simulink subsystem "State_Estimation_2WD_NO_REGEN"  (R2023b)
settings: Solver=VariableStepAuto  StartTime=0.0  StopTime=10.0  RelTol=1e-3
undefined symbols (not defined in the file): nI
libraries: dspstat3 x1
settings Model: Creator=Inver  LastModifiedBy=Inver

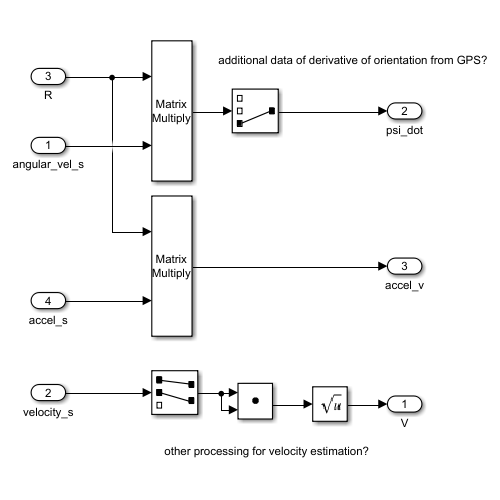
[thumbnail: Simulink's stored preview of the top-level diagram]
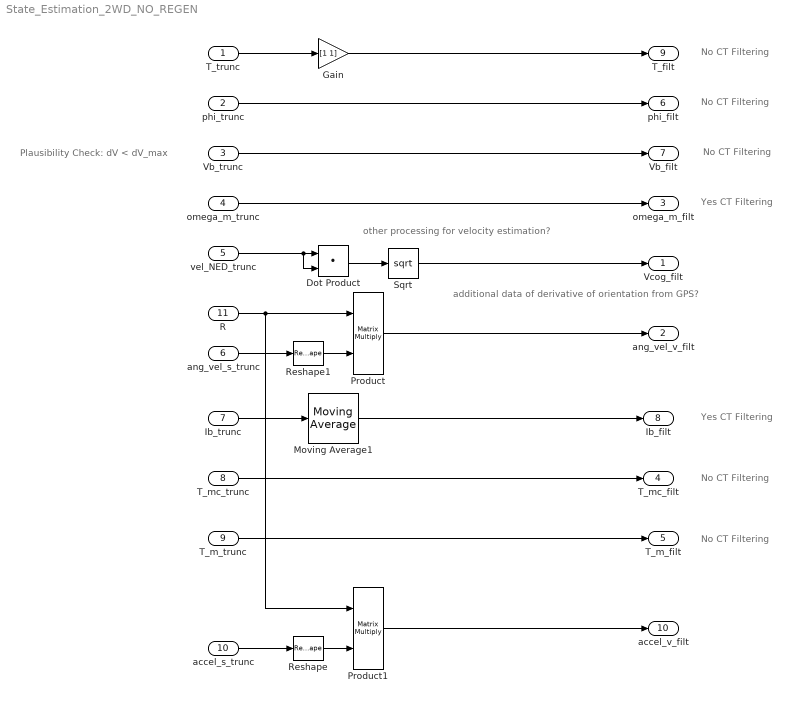
== system State_Estimation_2WD_NO_REGEN ==
  note: No CT Filtering
  note: Yes CT Filtering
  note: No CT Filtering
  note: No CT Filtering
  note: No CT Filtering
  note: No CT Filtering
  note: Plausibility Check: dV < dV_max
  note: Yes CT Filtering
  note: additional data of derivative of orientation from GPS?
  note: other processing for velocity estimation?
  T_trunc : Inport
  phi_trunc : Inport  Port=2
  Vb_trunc : Inport  Port=3
  omega_m_trunc : Inport  Port=4
  vel_NED_trunc : Inport  Port=5
  ang_vel_s_trunc : Inport  Port=6
  Ib_trunc : Inport  Port=7
  T_mc_trunc : Inport  Port=8
  T_m_trunc : Inport  Port=9
  accel_s_trunc : Inport  Port=10
  R : Inport  Port=11
  Dot Product : DotProduct  OutDataTypeStr=Inherit: Inherit via internal rule
  Gain : Gain  Gain=[1 1]
  Moving Average1 : dspstat3/Moving Average  Method=Sliding window  ForgettingFactorPort=off  SpecifyWindowLength=on  WindowLength=nI  OverlapLength=nI-1  AllowArbitraryInputLength=off  ForgettingFactor=0.9  SimulateUsing=Code generation
  Product : Product  Multiplication=Matrix(*)
  Product1 : Product  Multiplication=Matrix(*)
  Reshape : Reshape  OutputDimensions=[3 1]
  Reshape1 : Reshape  OutputDimensions=[3 1]
  Sqrt : Sqrt
  Vcog_filt : Outport
  ang_vel_v_filt : Outport  Port=2
  omega_m_filt : Outport  Port=3
  T_mc_filt : Outport  Port=4
  T_m_filt : Outport  Port=5
  phi_filt : Outport  Port=6
  Vb_filt : Outport  Port=7
  Ib_filt : Outport  Port=8
  T_filt : Outport  Port=9
  accel_v_filt : Outport  Port=10
  wires:
  accel_s_trunc/1 -> Reshape/1
  T_trunc/1 -> Gain/1
  T_mc_trunc/1 -> T_mc_filt/1
  T_m_trunc/1 -> T_m_filt/1
  Moving Average1/1 -> Ib_filt/1
  Ib_trunc/1 -> Moving Average1/1
  Vb_trunc/1 -> Vb_filt/1
  phi_trunc/1 -> phi_filt/1
  omega_m_trunc/1 -> omega_m_filt/1
  Sqrt/1 -> Vcog_filt/1
  vel_NED_trunc/1 -> Dot Product/1, Dot Product/2
  Dot Product/1 -> Sqrt/1
  Product/1 -> ang_vel_v_filt/1
  ang_vel_s_trunc/1 -> Reshape1/1
  Gain/1 -> T_filt/1
  R/1 -> Product1/1, Product/1
  Reshape/1 -> Product1/2
  Reshape1/1 -> Product/2
  Product1/1 -> accel_v_filt/1
